simulink model "SmAHTR_r1_PITTRTNUKE"  (R2014a)
settings: Solver=ode4  StartTime=0.0  StopTime=250  FixedStep=.001  RelTol=1e-3
PreLoadFcn:
  | load DarkLowerCoeffs
  | load DarkMiddleCoeffs
  | load DarkUpperCoeffs
  | load breaks
values from neighbouring files (symbols this model uses):
  alpha = [ -2.61*pcm -0.53*pcm ]    [SmAHTR_Spatial_Kinetics.m]
  breaks = DarkLowerBreaks    [SmAHTR_Spatial_Kinetics.m]
  cpc = 2414    [SmAHTR_Spatial_Kinetics.m]
  cpp = 2414    [SmAHTR_Spatial_Kinetics.m]
  DarkLowerCoeffs = ppDarkLower.coefs    [SmAHTR_Spatial_Kinetics.m]
  DarkMiddleCoeffs = ppDarkMiddle.coefs    [SmAHTR_Spatial_Kinetics.m]
  DarkRodWorthInserted = -3*Beta    (= -0.00489)    [SmAHTR_Spatial_Kinetics.m]
  DarkUpperCoeffs = ppDarkUpper.coefs    [SmAHTR_Spatial_Kinetics.m]
  delta_t = 1 / sensor_sampling_rate    (= 0.001)    [HeatExchanger_ps.m]    (also in steady_data_76rssi_30_1.mat = 0.1; steady_data_76rssi_40.mat = 0.1; steady_data_76rssi_iter.mat = 0.1; steady_data_76rssi_iter_reduce.mat = 0.1)
  Kc1 = 1/(rho_secondary*V_secondary)    (= 0.00032726218348)    [SmAHTR_Spatial_Kinetics.m]
  Kc2 = (h_secondary*A)/(cps*rho_secondary*V_secondary)    (= 1.23242359038)    [SmAHTR_Spatial_Kinetics.m]
  Kh1 = 1/(rho_primary*V_primary)    (= 0.000447917898441)    [SmAHTR_Spatial_Kinetics.m]
  Kh2 = (h_primary*A)/(cpp*rho_primary*V_primary)    (= 1.29038206968)    [SmAHTR_Spatial_Kinetics.m]
  Kw1 = h_primary    (= 23800)    [SmAHTR_Spatial_Kinetics.m]
  Kw2 = h_secondary    (= 24500)    [SmAHTR_Spatial_Kinetics.m]
  Kw3 = A/(rho_tube*cpw*V_tube)    (= 0.000122049789882)    [SmAHTR_Spatial_Kinetics.m]
  L1 = .0124    (= 0.0124)    [SmAHTR_Spatial_Kinetics.m]
  L2 = .0305    (= 0.0305)    [SmAHTR_Spatial_Kinetics.m]
  rcp_activatetime = 20    [SmAHTR_Spatial_Kinetics.m]
  rcpt = 0.1    [SmAHTR_Spatial_Kinetics.m]
  SaltVaultICs = -AtempSALT\btempSALT*u0    [SmAHTR_Spatial_Kinetics.m]
  Tp_i = 700    [SmAHTR_Spatial_Kinetics.m]
  Ts_i = 600    [SmAHTR_Spatial_Kinetics.m]
  Tw_i = 650    [SmAHTR_Spatial_Kinetics.m]
  xfc0 = -Atemp\btemp*u0    [SmAHTR_Spatial_Kinetics.m]
libraries: powerlib_meascontrol x9, simulink x3
(part 2 of 2)

== matlab function SmAHTR_r1_PITTRTNUKE/Reactor Kinetics and Thermal Hydraulics/Reactor Thermal-Hydraulics Zone 1/MATLAB Function ==
  data: m_dot input; Q_rx input; constants input; y output; T_c input; x input; x_dot output
function [y,x_dot] =FuelCoolantHX(m_dot,Q_rx,constants,T_c,x)

cpc=constants(1);
cpf=constants(2);
mc=constants(3);
mf=constants(4);
uh=constants(5);
Ar=constants(6);

A=[-(uh*Ar)/(mf*cpf), (uh*Ar)/(mf*cpf); (uh*Ar)/(mc*cpc), -(uh*Ar)/(mc*cpc)-(2*m_dot)/mc];

K=125000000/3;

b=[K/(mf*cpf), 0; 0 2*m_dot/mc];

u=[Q_rx; T_c];

x_dot=A*x+b*u;

C=[1 0; 0 1; 0 2];
D=[0 0;0 0; 0 -1];

y=C*x+D*u;

return

== matlab function SmAHTR_r1_PITTRTNUKE/Reactor Kinetics and Thermal Hydraulics/Reactor Thermal-Hydraulics Zone 3/MATLAB Function ==
  data: m_dot input; Q_rx input; constants input; y output; T_c input; x input; x_dot output
function [y,x_dot] =FuelCoolantHX(m_dot,Q_rx,constants,T_c,x)

cpc=constants(1);
cpf=constants(2);
mc=constants(3);
mf=constants(4);
uh=constants(5);
Ar=constants(6);

A=[-(uh*Ar)/(mf*cpf), (uh*Ar)/(mf*cpf); (uh*Ar)/(mc*cpc), -(uh*Ar)/(mc*cpc)-(2*m_dot)/mc];

K=125000000/3;

b=[K/(mf*cpf), 0; 0 2*m_dot/mc];

u=[Q_rx; T_c];

x_dot=A*x+b*u;

C=[1 0; 0 1; 0 2];
D=[0 0;0 0; 0 -1];

y=C*x+D*u;

return

== matlab function SmAHTR_r1_PITTRTNUKE/Reactor Kinetics and Thermal Hydraulics/Zone 2 Kinetics1 ==
  data: PROMPTN1 input; PROMPTN2 input; DELAYEDN1 input; DELAYEDN2 input; pkeparams input; rho_temp input; x input; y output; xdot output
function [y,xdot] = Zone2Kinetics(PROMPTN1,PROMPTN2,DELAYEDN1,DELAYEDN2,pkeparams,rho_temp,x)
%#codegen
% 
% K=reshape(Lcoupling,12,12); %Reshape the coupling matrix
% 
% %Unpackage the prompt and delayed neutron sources
% 
% %Prompt neuton unpackaging
N1 = PROMPTN1;
N2 = PROMPTN2;
% N2 = PROMPTN(2); N3 = PROMPTN(3); N4 = PROMPTN(4);
% N5 = PROMPTN(5); N6 = PROMPTN(6); N7 = PROMPTN(7);
% N8 = PROMPTN(8); N9 = PROMPTN(9); N10 = PROMPTN(10);
% N11 = PROMPTN(11); N12 = PROMPTN(12);
% 
% %Delayed neutron unpackaging
D1 = DELAYEDN1;
D2 = DELAYEDN2;
% D2 = DELAYEDN(2); D3 = DELAYEDN(3); D4 = DELAYEDN(4);
% D5 = DELAYEDN(5); D6 = DELAYEDN(6); D7 = DELAYEDN(7);
% D8 = DELAYEDN(8); D9 = DELAYEDN(9); D10 = DELAYEDN(10);
% D11 = DELAYEDN(11); D12 = DELAYEDN(12);

%PKE parameter load
Beta = pkeparams(1); B1 = pkeparams(2); B2 = pkeparams(3); B3 = pkeparams(4);
B4 = pkeparams(5); B5 = pkeparams(6); B6 = pkeparams(7); L1 = pkeparams(8);
L2 = pkeparams(9); L3 = pkeparams(10); L4 = pkeparams(11); L5 = pkeparams(12);
L6 = pkeparams(13); lambda = pkeparams(14);

%Reactivity coupling effects from other zones
alpha = (1-Beta)/lambda;
% 
rho_1 = lambda*0.005*(alpha*(N1/x(1))+0.005*(1/lambda)*D1/x(1));
rho_2 = lambda*0.005*(alpha*(N2/x(1))+0.005*(1/lambda)*D2/x(1));
% rho_3 = lambda*K(11,3)*(alpha*(N3/x(1))+(1/lambda)*D3/x(1));
% rho_4 = lambda*K(11,4)*(alpha*(N4/x(1))+(1/lambda)*D4/x(1));
% rho_5 = lambda*K(11,5)*(alpha*(N5/x(1))+(1/lambda)*D5/x(1));
% rho_6 = lambda*K(11,6)*(alpha*(N6/x(1))+(1/lambda)*D6/x(1));
% rho_7 = lambda*K(11,7)*(alpha*(N7/x(1))+(1/lambda)*D7/x(1));
% rho_8 = lambda*K(11,8)*(alpha*(N8/x(1))+(1/lambda)*D8/x(1));
% rho_9 = lambda*K(11,9)*(alpha*(N9/x(1))+(1/lambda)*D9/x(1));
% rho_10 = lambda*K(11,10)*(alpha*(N10/x(1))+(1/lambda)*D10/x(1));
% % rho_11 = lambda*K(11,11)*(alpha*(N11/x(1))+(1/lambda)*D11/x(1));
% rho_12 = lambda*K(11,12)*(alpha*(N12/x(1))+(1/lambda)*D12/x(1));
% 
% %Total reactivity
% 
% rho_t=rho_temp+rho_1+rho_2+rho_3+rho_4+rho_5+rho_6+rho_7+rho_8+rho_9+rho_10+rho_12;

%Reactor Point Kinetics State Equation
rho_t=rho_temp+rho_1+rho_2;

A = [(rho_t-Beta)/lambda L1/lambda L2/lambda;...
    B1 -L1 0;...
    B2 0 -L2];

C = [1 0 0;...
    0 L1 L2];

xdot = zeros(3,1,'double');
xdot = A*x;
y = zeros(2,1,'double');
y = C*x;

return

== matlab function SmAHTR_r1_PITTRTNUKE/Reactor Kinetics and Thermal Hydraulics/MATLAB Function ==
  data: DarkLowerCoeffs input; RodWorthLower output; DarkMiddleCoeffs input; DarkUpperCoeffs input; breaks input; RodWithdrawn input; RodWorthMiddle output; RodWorthUpper output
function [RodWorthLower,RodWorthMiddle,RodWorthUpper] = RodWorthIAEACurveFit(DarkLowerCoeffs,DarkMiddleCoeffs,DarkUpperCoeffs,breaks,...
    RodWithdrawn)

persistent L M U

for i = 1:length(breaks)-1
    if RodWithdrawn >= breaks(i) && RodWithdrawn < breaks(i+1)
        L = polyval(DarkLowerCoeffs(i,:),RodWithdrawn - breaks(i));
        M = polyval(DarkMiddleCoeffs(i,:),RodWithdrawn - breaks(i));
        U = polyval(DarkUpperCoeffs(i,:),RodWithdrawn - breaks(i));
        RodWorthLower = L;
        RodWorthMiddle = M;
        RodWorthUpper = U;
        return
    else
        L = 0;
        M = 0;
        U = 0;
        continue
    end
end

RodWorthLower = L;
RodWorthMiddle = M;
RodWorthUpper = U;

== matlab function SmAHTR_r1_PITTRTNUKE/Downcomer mixing dynamics/MATLAB Function ==
  data: a input; y output; b input; c input; d input; e input; f input; g input; z output
function [y,z] = fcn(a,b,c,d,e,f,g)
%#codegen

y=(b/a)*e+(c/a)*f+(d/a)*g;
z=b+c+d;

== matlab function SmAHTR_r1_PITTRTNUKE/Reactor Kinetics and Thermal Hydraulics/Reactor Thermal-Hydraulics Zone 2/MATLAB Function ==
  data: m_dot input; Q_rx input; constants input; y output; T_c input; x input; x_dot output
function [y,x_dot] =FuelCoolantHX(m_dot,Q_rx,constants,T_c,x)

cpc=constants(1);
cpf=constants(2);
mc=constants(3);
mf=constants(4);
uh=constants(5);
Ar=constants(6);

A=[-(uh*Ar)/(mf*cpf), (uh*Ar)/(mf*cpf); (uh*Ar)/(mc*cpc), -(uh*Ar)/(mc*cpc)-(2*m_dot)/mc];

K=125000000/3;

b=[K/(mf*cpf), 0; 0 2*m_dot/mc];

u=[Q_rx; T_c];

x_dot=A*x+b*u;

C=[1 0; 0 1; 0 2];
D=[0 0;0 0; 0 -1];

y=C*x+D*u;

return

== matlab function SmAHTR_r1_PITTRTNUKE/MATLAB Function ==
  data: m1 input; SHX_massflow output; m2 input; m3 input; T1 input; T2 input; T3 input; SHX_temp output
function [SHX_massflow,SHX_temp] = SaltVaultMassAveraging(m1,m2,m3,T1,T2,T3)

SHX_massflow=m1+m2+m3;

SHX_temp=(m1/SHX_massflow)*T1+(m2/SHX_massflow)*T2+(m3/SHX_massflow)*T3;

return

== matlab function SmAHTR_r1_PITTRTNUKE/MATLAB Function1 ==
  data: y output; Tt_o output; Tc_o output; xdot output; Tc_i input; Tt_i input; mdot input; constants input; x input

function [y,Tt_o,Tc_o,xdot]=BraytonCycle(Tc_i,Tt_i,mdot,constants,x)


% u=[Tc_i;Tt_i];


eta_C=constants(1); %compressor efficiency
eta_T=constants(2); %turbine efficiency
r=constants(3); %isotropic pressure ratio
cpCO2Turbine=constants(4); %specific heat capacity of gas (which is air)
cpCO2Compressor=constants(5);
% rhoCO2=constants(6);
tau_t=constants(7); %Compressor-turbine time constant

Tc_o=(Tc_i+273)*((r-1)/eta_C+1)-273; %Compressor outlet temperature
Tt_o=(Tt_i+273)*(1-eta_T*(1-(1/r)))-273; %Turbine outlet temperature

Pt=mdot*cpCO2Turbine*(Tt_i-Tt_o); %Turbine power
Pc=mdot*cpCO2Compressor*(Tc_o-Tc_i); %Compressor power

u=Pt-Pc; %Preliminary input to state space model;

%Our state is the mechanical / shaft power produced 

A=-1/tau_t; 
B=1/tau_t;
C=1;
D=0;

%We are calcuating only the net mechanical output power, for now.
xdot=A*x+B*u;
y=C*x+D*u;


return

== matlab function SmAHTR_r1_PITTRTNUKE/Salt Vault/Salt Vault ==
  data: y output; mdots input; x_dot output; mdott input; T_s1 input; T_t1 input; constants input; Tamb input; x input
function [y,x_dot] = SaltVaultStateSpace(mdots,mdott,T_s1,T_t1,constants,Tamb,x)

V_secondary=constants(1);
rho_secondary=constants(2);
cps=constants(3);
rhoCO2=constants(4);
m1=V_secondary*rho_secondary;
c1=cps;
m2=708; %Supercritical CO2 mass (TBD)
c2=1121;   %Supercritical CO2 specific heat (TBD)
h1=3400*7;  %Primary side of salt vault (secondary salt) effective heat transfer coefficient
h2=10000*3; %Supercritical CO2-side effective heat transfer coefficient (TBD)
ms=600000; %Mass of salt
cs=cps;    %Specific heat of salt
Area=292;

%Conditionally-implemented heat sink for salt vault temperature limit
    if x(2)>=540
        UA_thresh=5000000;
    else
        UA_thresh=0;
    end


u=[T_s1;Tamb;T_t1];

A=[-mdots/m1-h1*Area/(m1*c1), h1*Area/(m1*c1), 0;...
    h1*Area/(ms*cs), -h1*Area/(ms*cs)-h2*Area/(ms*cs)-(1*20000*pi())/(ms*cs)-UA_thresh/(ms*cs), h2*Area/(ms*cs);...
    0,h2*Area/(m2*c2), -mdott/m2-h2*Area/(m2*c2)];

b=[mdots/m1 0 0;0 (1*20000*pi())/(ms*cs)+UA_thresh/(ms*cs) 0; 0 0 mdott/m2];

C=[1 0 0;0 1 0;0 0 1];

D=zeros(3,3);

x_dot=A*x+b*u;

y=C*x+D*u;

return

== matlab function SmAHTR_r1_PITTRTNUKE/Reactor Kinetics and Thermal Hydraulics/Zone 3 Kinetics1 ==
  data: PROMPTN1 input; PROMPTN2 input; DELAYEDN1 input; DELAYEDN2 input; pkeparams input; rho_temp input; x input; y output; xdot output
function [y,xdot] = Zone3Kinetics(PROMPTN1,PROMPTN2,DELAYEDN1,DELAYEDN2,pkeparams,rho_temp,x)
%#codegen
% 
% K=reshape(Lcoupling,12,12); %Reshape the coupling matrix
% 
% %Unpackage the prompt and delayed neutron sources
% 
% %Prompt neuton unpackaging
N1 = PROMPTN1;
N2 = PROMPTN2;
% N2 = PROMPTN(2); N3 = PROMPTN(3); N4 = PROMPTN(4);
% N5 = PROMPTN(5); N6 = PROMPTN(6); N7 = PROMPTN(7);
% N8 = PROMPTN(8); N9 = PROMPTN(9); N10 = PROMPTN(10);
% N11 = PROMPTN(11); N12 = PROMPTN(12);
% 
% %Delayed neutron unpackaging
D1 = DELAYEDN1;
D2 = DELAYEDN2;
% D2 = DELAYEDN(2); D3 = DELAYEDN(3); D4 = DELAYEDN(4);
% D5 = DELAYEDN(5); D6 = DELAYEDN(6); D7 = DELAYEDN(7);
% D8 = DELAYEDN(8); D9 = DELAYEDN(9); D10 = DELAYEDN(10);
% D11 = DELAYEDN(11); D12 = DELAYEDN(12);

%PKE parameter load
Beta = pkeparams(1); B1 = pkeparams(2); B2 = pkeparams(3); B3 = pkeparams(4);
B4 = pkeparams(5); B5 = pkeparams(6); B6 = pkeparams(7); L1 = pkeparams(8);
L2 = pkeparams(9); L3 = pkeparams(10); L4 = pkeparams(11); L5 = pkeparams(12);
L6 = pkeparams(13); lambda = pkeparams(14);

%Reactivity coupling effects from other zones
alpha = (1-Beta)/lambda;
% 
rho_1 = lambda*0.002*(alpha*(N1/x(1))+0.002*(1/lambda)*D1/x(1));
rho_2 = lambda*0.005*(alpha*(N2/x(1))+0.005*(1/lambda)*D2/x(1));
% rho_3 = lambda*K(11,3)*(alpha*(N3/x(1))+(1/lambda)*D3/x(1));
% rho_4 = lambda*K(11,4)*(alpha*(N4/x(1))+(1/lambda)*D4/x(1));
% rho_5 = lambda*K(11,5)*(alpha*(N5/x(1))+(1/lambda)*D5/x(1));
% rho_6 = lambda*K(11,6)*(alpha*(N6/x(1))+(1/lambda)*D6/x(1));
% rho_7 = lambda*K(11,7)*(alpha*(N7/x(1))+(1/lambda)*D7/x(1));
% rho_8 = lambda*K(11,8)*(alpha*(N8/x(1))+(1/lambda)*D8/x(1));
% rho_9 = lambda*K(11,9)*(alpha*(N9/x(1))+(1/lambda)*D9/x(1));
% rho_10 = lambda*K(11,10)*(alpha*(N10/x(1))+(1/lambda)*D10/x(1));
% % rho_11 = lambda*K(11,11)*(alpha*(N11/x(1))+(1/lambda)*D11/x(1));
% rho_12 = lambda*K(11,12)*(alpha*(N12/x(1))+(1/lambda)*D12/x(1));
% 
% %Total reactivity
% 
% rho_t=rho_temp+rho_1+rho_2+rho_3+rho_4+rho_5+rho_6+rho_7+rho_8+rho_9+rho_10+rho_12;

%Reactor Point Kinetics State Equation
rho_t=rho_temp+rho_1+rho_2;

A = [(rho_t-Beta)/lambda L1/lambda L2/lambda;...
    B1 -L1 0;...
    B2 0 -L2];

C = [1 0 0;...
    0 L1 L2];

xdot = zeros(3,1,'double');
xdot = A*x;
y = zeros(2,1,'double');
y = C*x;

return

== matlab function SmAHTR_r1_PITTRTNUKE/Reactor Kinetics and Thermal Hydraulics/Zone 1 Kinetics1 ==
  data: PROMPTN1 input; PROMPTN2 input; DELAYEDN1 input; DELAYEDN2 input; pkeparams input; rho_temp input; x input; y output; xdot output
function [y,xdot] = Zone1Kinetics(PROMPTN1,PROMPTN2,DELAYEDN1,DELAYEDN2,pkeparams,rho_temp,x)
%#codegen
% 
% K=reshape(Lcoupling,12,12); %Reshape the coupling matrix
% 
% %Unpackage the prompt and delayed neutron sources
% 
% %Prompt neuton unpackaging
N1 = PROMPTN1;
N2 = PROMPTN2;
% N2 = PROMPTN(2); N3 = PROMPTN(3); N4 = PROMPTN(4);
% N5 = PROMPTN(5); N6 = PROMPTN(6); N7 = PROMPTN(7);
% N8 = PROMPTN(8); N9 = PROMPTN(9); N10 = PROMPTN(10);
% N11 = PROMPTN(11); N12 = PROMPTN(12);
% 
% %Delayed neutron unpackaging
D1 = DELAYEDN1;
D2 = DELAYEDN2;
% D2 = DELAYEDN(2); D3 = DELAYEDN(3); D4 = DELAYEDN(4);
% D5 = DELAYEDN(5); D6 = DELAYEDN(6); D7 = DELAYEDN(7);
% D8 = DELAYEDN(8); D9 = DELAYEDN(9); D10 = DELAYEDN(10);
% D11 = DELAYEDN(11); D12 = DELAYEDN(12);

%PKE parameter load
Beta = pkeparams(1); B1 = pkeparams(2); B2 = pkeparams(3); B3 = pkeparams(4);
B4 = pkeparams(5); B5 = pkeparams(6); B6 = pkeparams(7); L1 = pkeparams(8);
L2 = pkeparams(9); L3 = pkeparams(10); L4 = pkeparams(11); L5 = pkeparams(12);
L6 = pkeparams(13); lambda = pkeparams(14);

%Reactivity coupling effects from other zones
alpha = (1-Beta)/lambda;
% 
rho_1 = lambda*0.005*(alpha*(N1/x(1))+0.005*(1/lambda)*D1/x(1));
rho_2 = lambda*0.002*(alpha*(N2/x(1))+0.002*(1/lambda)*D2/x(1));
% rho_3 = lambda*K(11,3)*(alpha*(N3/x(1))+(1/lambda)*D3/x(1));
% rho_4 = lambda*K(11,4)*(alpha*(N4/x(1))+(1/lambda)*D4/x(1));
% rho_5 = lambda*K(11,5)*(alpha*(N5/x(1))+(1/lambda)*D5/x(1));
% rho_6 = lambda*K(11,6)*(alpha*(N6/x(1))+(1/lambda)*D6/x(1));
% rho_7 = lambda*K(11,7)*(alpha*(N7/x(1))+(1/lambda)*D7/x(1));
% rho_8 = lambda*K(11,8)*(alpha*(N8/x(1))+(1/lambda)*D8/x(1));
% rho_9 = lambda*K(11,9)*(alpha*(N9/x(1))+(1/lambda)*D9/x(1));
% rho_10 = lambda*K(11,10)*(alpha*(N10/x(1))+(1/lambda)*D10/x(1));
% % rho_11 = lambda*K(11,11)*(alpha*(N11/x(1))+(1/lambda)*D11/x(1));
% rho_12 = lambda*K(11,12)*(alpha*(N12/x(1))+(1/lambda)*D12/x(1));
% 
% %Total reactivity
% 
% rho_t=rho_temp+rho_1+rho_2+rho_3+rho_4+rho_5+rho_6+rho_7+rho_8+rho_9+rho_10+rho_12;

%Reactor Point Kinetics State Equation
rho_t=rho_temp+rho_1+rho_2;

A = [(rho_t-Beta)/lambda L1/lambda L2/lambda;...
    B1 -L1 0;...
    B2 0 -L2];

C = [1 0 0;...
    0 L1 L2];

xdot = zeros(3,1,'double');
xdot = A*x;
y = zeros(2,1,'double');
y = C*x;

return

== matlab function SmAHTR_r1_PITTRTNUKE/Tossim Up1 ==
  data: ymea1 output; ymea input; ydelay output; ydelay_global data_store_memory; ynetwork_delay output; counter_global data_store_memory
function [ymea1, ydelay, ynetwork_delay]  = Tossim_block(ymea)

% Inputs:
% ymea: measurement from structure

% Outputs:
% ymea1: measurement output
% ydelay: delay traces

persistent delay1 % delay trace
persistent i  % count
persistent last_emergency_instance RetransCounter
persistent network_array
global ydelay_global
global counter_global

iterations = 200002;



% allow these matlab functions to be used in Embedded Matlab block
eml.extrinsic('python');
eml.extrinsic('num2str');
eml.extrinsic('str2num');
eml.extrinsic('delay_summary');
eml.extrinsic('disp');
%eml.extrinsic('ps_aggregation');
eml.extrinsic('ps_text');
eml.extrinsic('for');
eml.extrinsic('end');
eml.extrinsic('fgets');
eml.extrinsic('fopen');

if isempty(i)
    i = 0;
    
    % read "network_error_delay.txt" file
    network_array= zeros(iterations, 18);
    text = fopen('noError.txt');

    result = fgets(text);
    %disp(result);

    %network_array(1, :) = str2num(result);
    line_num=1;
    while ischar(result)
        if( line_num <=iterations)
            network_array(line_num, :) = str2num(result);
            result = fgets(text);
        else
            break;
        end

        line_num = line_num+1;

    end
    fclose(text);
    %disp(network_array);
end

i = i + 1;
%No, delay of L1H, delay of L2H, delay of L2, delay of LRL, delay of LRH£¬delay of L1H, delay of L2H, delay of L2, delay of LRL, delay of LRH

ydelay = [1 0 0 0 0 0 0 0 0 0]'; 
ynetwork_delay = [0, 0, 0, 0, 0, 0, 0, 0, 0]';

emergency_instance = ymea';

%call_count = 56; % number of slots + 1 (i.e., number of client calls made + 1) per TDMA schedule, +1 to have full 53 slots after %
%[resultz] = ps_aggregation(call_count);
%[resultz] = ps_text(i);
%disp(network_array);
resultz = network_array(i, :);
%resultz

%end_to_end_delivery_result_aggregated = sum(resultz);

%disp('end_to_end_delivery_result_aggregated')
%disp(end_to_end_delivery_result_aggregated)

[delay] = delay_summary(resultz);
ydelay = delay';

[network_delay] = network_delay_summary(resultz);
ynetwork_delay=network_delay';

disp('i');
disp(i);

last_emergency_instance = ymea';
delay1 = ydelay;


ymea1 = [0 0 0 0 0 0 0 0 0]'; %9 sensors
ymea1 = ymea;


for i_yg = 1:10
    ydelay_global(i_yg, 1) = ydelay(i_yg, 1);
end

%disp('Plant 1, TOSSIM Uplink Block, is called');
counter_global = counter_global + 1;

== matlab function SmAHTR_r1_PITTRTNUKE/Delayed Data Up2 ==
  data: yout input; ydelay input; yout_delay output; structure parameter
function yout_delay   = delay_block(yout,ydelay, structure)

% Inputs: 
% yout: measurements output
% ydelay: delay traces
% structure: other necessary information 
% Inputs: 
% yout: measurements output
% ydelay: delay traces

% Outputs:
% yout_delay: delayed measurements output for controller
persistent  i yin_d 
persistent yin delay yin_all num
eml.extrinsic('disp');

% sennum=5;  %number of the sensors
step_count = 800000; %step_count

% initialize parameters
if isempty(yin)
    i = structure.i;
    yin = structure.yin;
    yin_d = structure.yin_d; 
    yin_all = zeros(step_count+1,9); %zeros (step count, sensor number)
    
    delay = zeros(1,9+1);         %initialized
    delay = ydelay';
    
    num = 0;
end
 

num = num+1;   

%get delay information 
% delay=zeros(1,10+1); 
delay=ydelay';

%get value from "yout" input
for kk = 1:3
    yin_all(num,kk) = yout(kk); %offset=5
end    
    
%generate output value according to delay    
for j=1:3
    if delay(1,j+1)~=88
        yin(j) = yin_all(num,j);  %packet receive
    else
        if num>1 
%             yin(j)=0;  %if lost, set it to zero
             yin(j)=yin_all(num-1,j); %if lost, set it to previous value
             yin_all(num,j)=yin_all(num-1,j);
        end        
    end
end


yin_d = yin';

yout_delay = yin_d;


% disp('plant2');

% yout_delay'
i = i+1;


%yout_delay;
% disp('yout_delay');
% disp(yout_delay');
% disp('i')
% disp(i)
